simulink model "TorqueVectoring"  (R2023b)
settings: Solver=VariableStepAuto  StartTime=0.0  StopTime=25  FixedStep=1e-3  RelTol=1e-1  AbsTol=1e-3
libraries: simulink x7, autolibshared x5, fuzblock x5, vehdynlibviscommon x1, sim3dlib x1, sim3dautolib x1
(part 6 of 6)

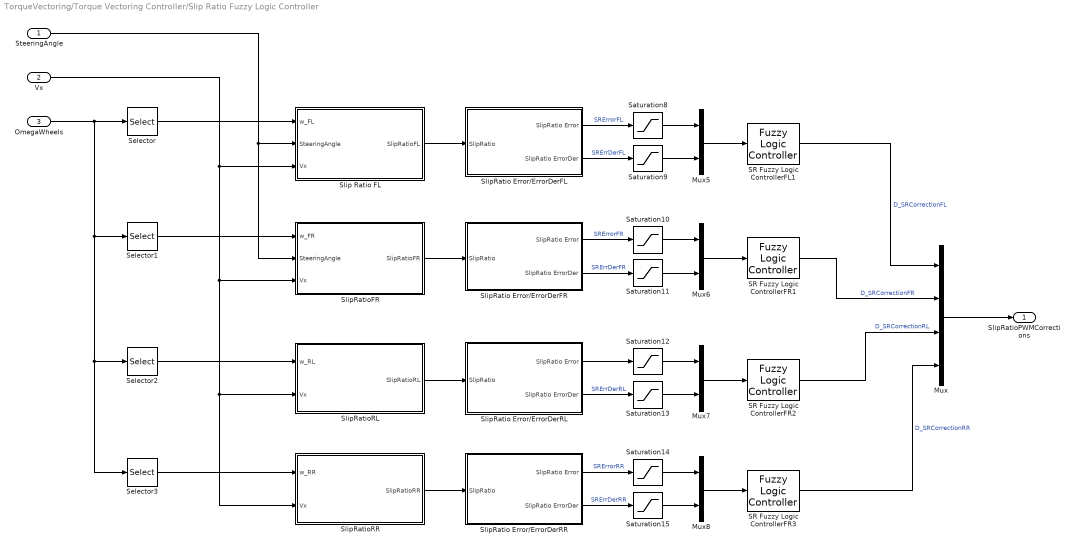
== system TorqueVectoring/Torque Vectoring Controller/Slip Ratio Fuzzy Logic Controller ==
  SteeringAngle : Inport
  Vx : Inport  Port=2
  OmegaWheels : Inport  Port=3
  Mux : Mux
  Mux{5..8} (4 alike) : Mux  Inputs=2
  SR Fuzzy Logic ControllerFL1 : fuzblock/Fuzzy Logic  Controller  FIS='SRfuzzyrules.fis'  OutputSampleNumber=101  DataType=double  FuzzifiedInputs=off  RuleFiringStrengths=off  RuleOutputs=off  AggregatedOutputs=off  SimulateUsing=Interpreted execution  OutOfRangeInputValueMessage=warning  NoRuleFiredMessage=warning  EmptyOutputFuzzySetMessage=warning
  SR Fuzzy Logic ControllerFR1 : fuzblock/Fuzzy Logic  Controller  FIS='SRfuzzyrules.fis'  OutputSampleNumber=101  DataType=double  FuzzifiedInputs=off  RuleFiringStrengths=off  RuleOutputs=off  AggregatedOutputs=off  SimulateUsing=Interpreted execution  OutOfRangeInputValueMessage=warning  NoRuleFiredMessage=warning  EmptyOutputFuzzySetMessage=warning
  SR Fuzzy Logic ControllerFR2 : fuzblock/Fuzzy Logic  Controller  FIS='SRfuzzyrules.fis'  OutputSampleNumber=101  DataType=double  FuzzifiedInputs=off  RuleFiringStrengths=off  RuleOutputs=off  AggregatedOutputs=off  SimulateUsing=Interpreted execution  OutOfRangeInputValueMessage=warning  NoRuleFiredMessage=warning  EmptyOutputFuzzySetMessage=warning
  SR Fuzzy Logic ControllerFR3 : fuzblock/Fuzzy Logic  Controller  FIS='SRfuzzyrules.fis'  OutputSampleNumber=101  DataType=double  FuzzifiedInputs=off  RuleFiringStrengths=off  RuleOutputs=off  AggregatedOutputs=off  SimulateUsing=Interpreted execution  OutOfRangeInputValueMessage=warning  NoRuleFiredMessage=warning  EmptyOutputFuzzySetMessage=warning
  Saturation{8,10,12,14} (4 alike) : Saturate  UpperLimit=30  LowerLimit=-30
  Saturation{9,11,13,15} (4 alike) : Saturate  UpperLimit=3e4  LowerLimit=-3e4
  Selector : Selector  InputPortWidth=4  IndexOptions=Index vector (dialog)  Indices=1  OutputSizes=1
  Selector1 : Selector  InputPortWidth=4  IndexOptions=Index vector (dialog)  Indices=2  OutputSizes=1
  Selector2 : Selector  InputPortWidth=4  IndexOptions=Index vector (dialog)  Indices=3  OutputSizes=1
  Selector3 : Selector  InputPortWidth=4  IndexOptions=Index vector (dialog)  Indices=4  OutputSizes=1
  Slip Ratio FL : Subsystem
  SlipRatio Error/ErrorDerFL : Subsystem
  SlipRatio Error/ErrorDerFR : Subsystem
  SlipRatio Error/ErrorDerRL : Subsystem
  SlipRatio Error/ErrorDerRR : Subsystem
  SlipRatioFR : Subsystem
  SlipRatioRL : Subsystem
  SlipRatioRR : Subsystem
  SlipRatioPWMCorrections : Outport
  wires:
  Selector/1 -> Slip Ratio FL/1(w_FL)
  Selector1/1 -> SlipRatioFR/1(w_FR)
  Selector2/1 -> SlipRatioRL/1(w_RL)
  Selector3/1 -> SlipRatioRR/1(w_RR)
  Mux/1 -> SlipRatioPWMCorrections/1
  SteeringAngle/1 -> SlipRatioFR/2(SteeringAngle), Slip Ratio FL/2(SteeringAngle)
  Vx/1 -> SlipRatioRR/2(Vx), SlipRatioRL/2(Vx), SlipRatioFR/3(Vx), Slip Ratio FL/3(Vx)
  OmegaWheels/1 -> Selector3/1, Selector2/1, Selector1/1, Selector/1
  Slip Ratio FL/1(SlipRatioFL) -> SlipRatio Error/ErrorDerFL/1(SlipRatio)
  SlipRatioFR/1(SlipRatioFR) -> SlipRatio Error/ErrorDerFR/1(SlipRatio)
  SlipRatioRL/1(SlipRatioRL) -> SlipRatio Error/ErrorDerRL/1(SlipRatio)
  SlipRatioRR/1(SlipRatioRR) -> SlipRatio Error/ErrorDerRR/1(SlipRatio)
  Saturation9/1 -> Mux5/2
  Saturation8/1 -> Mux5/1
  Mux5/1 -> SR Fuzzy Logic ControllerFL1/1
  SR Fuzzy Logic ControllerFL1/1 -> Mux/1  "D_SRCorrectionFL"
  Mux6/1 -> SR Fuzzy Logic ControllerFR1/1
  Saturation10/1 -> Mux6/1
  Saturation11/1 -> Mux6/2
  SR Fuzzy Logic ControllerFR1/1 -> Mux/2  "D_SRCorrectionFR"
  Saturation13/1 -> Mux7/2
  Saturation12/1 -> Mux7/1
  Mux7/1 -> SR Fuzzy Logic ControllerFR2/1
  SR Fuzzy Logic ControllerFR2/1 -> Mux/3  "D_SRCorrectionRL"
  Mux8/1 -> SR Fuzzy Logic ControllerFR3/1
  Saturation14/1 -> Mux8/1
  Saturation15/1 -> Mux8/2
  SR Fuzzy Logic ControllerFR3/1 -> Mux/4  "D_SRCorrectionRR"
  SlipRatio Error/ErrorDerFL/1(SlipRatio Error) -> Saturation8/1  "SRErrorFL"
  SlipRatio Error/ErrorDerFL/2(SlipRatio ErrorDer) -> Saturation9/1  "SRErrDerFL"
  SlipRatio Error/ErrorDerFR/1(SlipRatio Error) -> Saturation10/1  "SRErrorFR"
  SlipRatio Error/ErrorDerFR/2(SlipRatio ErrorDer) -> Saturation11/1  "SRErrDerFR"
  SlipRatio Error/ErrorDerRL/1(SlipRatio Error) -> Saturation12/1
  SlipRatio Error/ErrorDerRL/2(SlipRatio ErrorDer) -> Saturation13/1  "SRErrDerRL"
  SlipRatio Error/ErrorDerRR/1(SlipRatio Error) -> Saturation14/1  "SRErrorRR"
  SlipRatio Error/ErrorDerRR/2(SlipRatio ErrorDer) -> Saturation15/1  "SRErrDerRR"

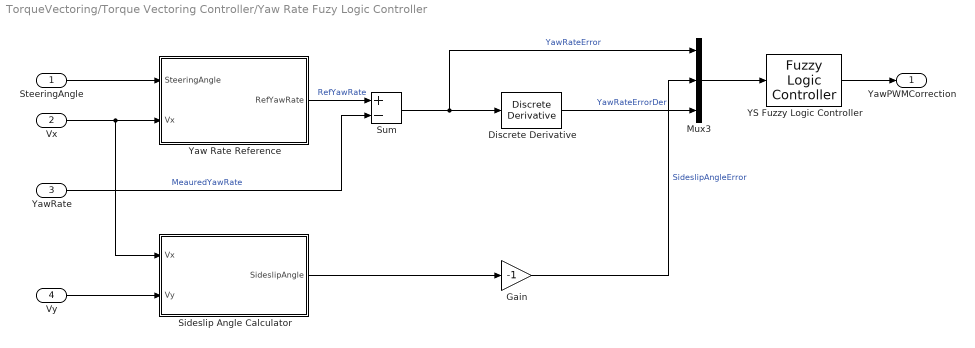
== system TorqueVectoring/Torque Vectoring Controller/Yaw Rate Fuzy Logic Controller ==
  SteeringAngle : Inport
  Vx : Inport  Port=2
  YawRate : Inport  Port=3
  Vy : Inport  Port=4
  Discrete Derivative : simulink/Discrete/Discrete Derivative  gainval=1.0  ICPrevScaledInput=0.0  OutMin=[]  OutMax=[]  OutDataType=fixdt(1, 16)  OutScaling=2^-10  DoSatur=off
  Gain : Gain  Gain=-1
  Mux3 : Mux  Inputs=3
  Sideslip Angle Calculator : Subsystem
  Sum : Sum  Inputs=+-
  YS Fuzzy Logic Controller : fuzblock/Fuzzy Logic  Controller  FIS='YSfuzzyrules.fis'  OutputSampleNumber=101  DataType=double  FuzzifiedInputs=off  RuleFiringStrengths=off  RuleOutputs=off  AggregatedOutputs=off  SimulateUsing=Interpreted execution  OutOfRangeInputValueMessage=warning  NoRuleFiredMessage=warning  EmptyOutputFuzzySetMessage=warning
  Yaw Rate Reference : Subsystem
  YawPWMCorrection : Outport
  wires:
  SteeringAngle/1 -> Yaw Rate Reference/1(SteeringAngle)
  YawRate/1 -> Sum/2  "MeauredYawRate"
  Sum/1 -> Discrete Derivative/1, Mux3/1  "YawRateError"
  Yaw Rate Reference/1(RefYawRate) -> Sum/1  "RefYawRate"
  Vx/1 -> Sideslip Angle Calculator/1(Vx), Yaw Rate Reference/2(Vx)
  Gain/1 -> Mux3/2  "SideslipAngleError"
  Discrete Derivative/1 -> Mux3/3  "YawRateErrorDer"
  Mux3/1 -> YS Fuzzy Logic Controller/1
  YS Fuzzy Logic Controller/1 -> YawPWMCorrection/1
  Vy/1 -> Sideslip Angle Calculator/2(Vy)
  Sideslip Angle Calculator/1(SideslipAngle) -> Gain/1

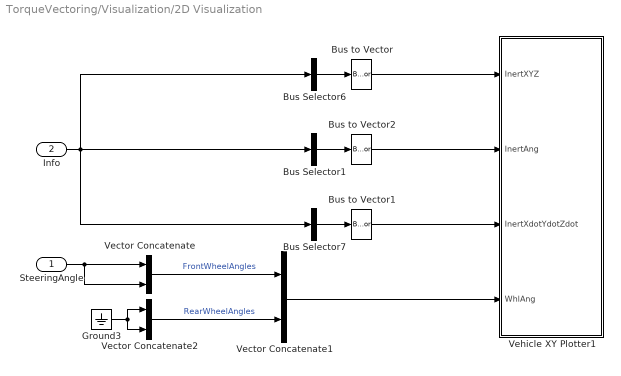
== system TorqueVectoring/Visualization/2D Visualization ==
  SteeringAngle : Inport
  Info : Inport  Port=2
  Bus Selector1 : BusSelector  OutputSignals=InertFrm.Cg.Ang.phi,InertFrm.Cg.Ang.theta,InertFrm.Cg.Ang.psi  OutputAsBus=on
  Bus Selector6 : BusSelector  OutputSignals=InertFrm.Geom.Disp.X,InertFrm.Geom.Disp.Y,InertFrm.Geom.Disp.Z  OutputAsBus=on
  Bus Selector7 : BusSelector  OutputSignals=InertFrm.Geom.Vel.Xdot,InertFrm.Geom.Vel.Ydot,InertFrm.Geom.Vel.Zdot  OutputAsBus=on
  Bus to Vector : BusToVector
  Bus to Vector1 : BusToVector
  Bus to Vector2 : BusToVector
  Ground3 : Ground
  Vector Concatenate : Concatenate
  Vector Concatenate1 : Concatenate
  Vector Concatenate2 : Concatenate
  Vehicle XY Plotter1 : Subsystem  mask(Vehicle XY Plotter){extRef=off, extStats=off, extTireF=off, a=0.175, b=0.175, w=0.2, figBorder=3, bufferSize=1024, velNorm=5, tireFNorm=1000, pltDT=0.2}
      mask prompts: extRef "Plot path reference, extRef"; extStats "Display speed, RPM and Gear"; extTireF "Display tire forces"; a "Distance to front axle from CG, a [m]:"; b "Distance to rear axle from CG, b [m]:"; w "Track width, w [m]:"; figBorder "Distance to figure borders, figBorder [m]:"; bufferSize "Path buffer sampe size, bufferSize []:"; velNorm "Velocity vector scaling, velNorm [m*s/m]:"; tireFNorm "Tire force vector scaling, tireFNorm [m/N]:"; pltDT "Plot update rate, pltDT [s]:"
      mask help:
      | This block will display a MATLAB figure which indicates the vehicle path, current position and heading velocity.
      | An optional path reference is also provided.
      mask init:
      | block = gcb;
      | if autoblkschecksimstopped(block)
      |     ParamNames = {'extRef';'extStats';'extTireF';'extTireF'};
      |     PortNames = {'RefXYZ';'Stats';'TireFx';'TireFy'};
      |     for idx=1:length(PortNames)
      |         InportOption  = {'built-in/Ground', [PortNames{idx}, ' Ground'];...
      |             'built-in/Inport',PortNames{idx}};
      |         if ~strcmp(get_param(block,ParamNames{idx}),'on')
      |             NewBlkHdl = autoblksreplaceblock(block, InportOption, 1);
      |             set_param(NewBlkHdl, 'ShowName', 'off');
      |         else
      |             autoblksreplaceblock(block, InportOption, 2);
      |         end
      |     end
      |     InportNames = {'InertXYZ';'InertAng';'InertXdotYdotZdot';'WhlAng';'RefXYZ';'Stats';'TireFx';'TireFy'};
      |     FoundNames = get_param(find_system(block, 'LookUnderMasks', 'all', 'SearchDepth', 1, 'FollowLinks', 'on', 'BlockType', 'Inport'), 'Name');
      |     [~,PortI] = intersect(InportNames, FoundNames);
      |     PortI = sort(PortI);
      |     for idx = 1:length(PortI)
      |         set_param([block, '/', InportNames{PortI(idx)}], 'Port', num2str(idx));
      |     end
      | end
      mask TypeOptions a: Vehicle XY Plotter/a
      mask TypeOptions b: Vehicle XY Plotter/b
      mask TypeOptions w: Vehicle XY Plotter/w
      mask TypeOptions figBorder: Vehicle XY Plotter/figBorder
      mask TypeOptions bufferSize: Vehicle XY Plotter/bufferSize
      mask TypeOptions velNorm: Vehicle XY Plotter/velNorm
      mask TypeOptions tireFNorm: Vehicle XY Plotter/tireFNorm
      mask DialogControl Container3 Prompt: Plot and Display Options
  wires:
  Vector Concatenate1/1 -> Vehicle XY Plotter1/4(WhlAng)
  Ground3/1 -> Vector Concatenate2/1, Vector Concatenate2/2
  Bus Selector6/1 -> Bus to Vector/1
  Vector Concatenate/1 -> Vector Concatenate1/1  "FrontWheelAngles"
  SteeringAngle/1 -> Vector Concatenate/2, Vector Concatenate/1
  Vector Concatenate2/1 -> Vector Concatenate1/2  "RearWheelAngles"
  Bus Selector7/1 -> Bus to Vector1/1
  Bus to Vector1/1 -> Vehicle XY Plotter1/3(InertXdotYdotZdot)
  Bus to Vector/1 -> Vehicle XY Plotter1/1(InertXYZ)
  Bus to Vector2/1 -> Vehicle XY Plotter1/2(InertAng)
  Bus Selector1/1 -> Bus to Vector2/1
  Info/1 -> Bus Selector6/1, Bus Selector7/1, Bus Selector1/1

== system TorqueVectoring/Plant/Wheel Front Left/DC Motor ==
  PWMVoltage : Inport
  w : Inport  Port=2
  Multiply : Gain  Gain=0.00402273
  Multiply1 : Gain  Gain=0.00006835
  Subtract : Sum  Inputs=+-
  Torque : Outport
  wires:
  Multiply1/1 -> Subtract/2
  PWMVoltage/1 -> Multiply/1
  Multiply/1 -> Subtract/1
  Subtract/1 -> Torque/1
  w/1 -> Multiply1/1

== system TorqueVectoring/Plant/Wheel Front Right/DC Motor ==
  PWMVoltage : Inport
  w : Inport  Port=2
  Multiply : Gain  Gain=0.00402273
  Multiply1 : Gain  Gain=0.00006835
  Subtract : Sum  Inputs=+-
  Torque : Outport
  wires:
  Multiply1/1 -> Subtract/2
  PWMVoltage/1 -> Multiply/1
  Multiply/1 -> Subtract/1
  Subtract/1 -> Torque/1
  w/1 -> Multiply1/1

== system TorqueVectoring/Plant/Wheel Rear Left/DC Motor ==
  PWMVoltage : Inport
  w : Inport  Port=2
  Multiply : Gain  Gain=0.00402273
  Multiply1 : Gain  Gain=0.00006835
  Subtract : Sum  Inputs=+-
  Torque : Outport
  wires:
  Multiply1/1 -> Subtract/2
  PWMVoltage/1 -> Multiply/1
  Multiply/1 -> Subtract/1
  Subtract/1 -> Torque/1
  w/1 -> Multiply1/1

== system TorqueVectoring/Plant/Wheel Rear Right/DC Motor ==
  PWMVoltage : Inport
  w : Inport  Port=2
  Multiply : Gain  Gain=0.00402273
  Multiply1 : Gain  Gain=0.00006835
  Subtract : Sum  Inputs=+-
  Torque : Outport
  wires:
  Multiply1/1 -> Subtract/2
  PWMVoltage/1 -> Multiply/1
  Multiply/1 -> Subtract/1
  Subtract/1 -> Torque/1
  w/1 -> Multiply1/1

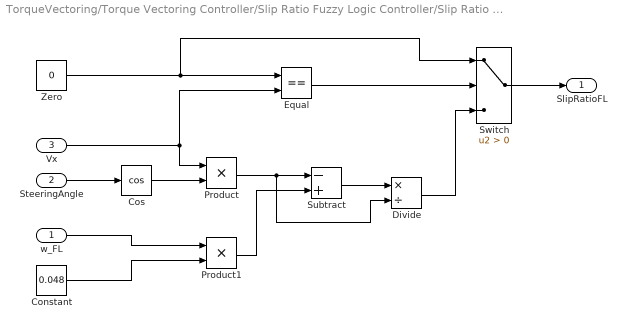
== system TorqueVectoring/Torque Vectoring Controller/Slip Ratio Fuzzy Logic Controller/Slip Ratio FL ==
  w_FL : Inport
  SteeringAngle : Inport  Port=2
  Vx : Inport  Port=3
  Constant : Constant  Value=0.048
  Cos : Trigonometry  Operator=cos
  Divide : Product  Inputs=*/
  Equal : RelationalOperator  Operator===  OutDataTypeStr=boolean  RndMeth=Simplest  InputSameDT=off
  Product : Product
  Product1 : Product
  Subtract : Sum  Inputs=-+
  Switch : Switch  Criteria=u2 > Threshold  SaturateOnIntegerOverflow=off  InputSameDT=off
  Zero : Constant  Value=0  OutDataTypeStr=Inherit: Inherit via back propagation
  SlipRatioFL : Outport
  wires:
  Constant/1 -> Product1/2
  SteeringAngle/1 -> Cos/1
  Product/1 -> Divide/2, Subtract/1
  Product1/1 -> Subtract/2
  Subtract/1 -> Divide/1
  Cos/1 -> Product/2
  w_FL/1 -> Product1/1
  Vx/1 -> Equal/2, Product/1
  Zero/1 -> Switch/1, Equal/1
  Equal/1 -> Switch/2
  Switch/1 -> SlipRatioFL/1
  Divide/1 -> Switch/3

== system TorqueVectoring/Torque Vectoring Controller/Slip Ratio Fuzzy Logic Controller/SlipRatio Error//ErrorDerFL ==
  SlipRatio : Inport
  Discrete Derivative : simulink/Discrete/Discrete Derivative  gainval=1.0  ICPrevScaledInput=0.0  OutMin=[]  OutMax=[]  OutDataType=fixdt(1, 16)  OutScaling=2^-10  DoSatur=off
  SlipRatioError1 : Sum  Inputs=+-
  SlipRatioRef1 : Subsystem
  SlipRatioToError1 : Subsystem
  SlipRatio Error : Outport
  SlipRatio ErrorDer : Outport  Port=2
  wires:
  SlipRatioToError1/1(SlipRatioToError) -> SlipRatioError1/2  "D_SRactual"
  SlipRatioRef1/1(SlipRatioRef) -> SlipRatioError1/1  "D_SRref"
  SlipRatioError1/1 -> SlipRatio Error/1, Discrete Derivative/1
  SlipRatio/1 -> SlipRatioToError1/1(SlipRatio), SlipRatioRef1/1(SlipRatio)
  Discrete Derivative/1 -> SlipRatio ErrorDer/1

== system TorqueVectoring/Torque Vectoring Controller/Slip Ratio Fuzzy Logic Controller/SlipRatio Error//ErrorDerFR ==
  SlipRatio : Inport
  Discrete Derivative1 : simulink/Discrete/Discrete Derivative  gainval=1.0  ICPrevScaledInput=0.0  OutMin=[]  OutMax=[]  OutDataType=fixdt(1, 16)  OutScaling=2^-10  DoSatur=off
  SlipRatioError1 : Sum  Inputs=+-
  SlipRatioRef1 : Subsystem
  SlipRatioToError1 : Subsystem
  SlipRatio Error : Outport
  SlipRatio ErrorDer : Outport  Port=2
  wires:
  SlipRatio/1 -> SlipRatioToError1/1(SlipRatio), SlipRatioRef1/1(SlipRatio)
  SlipRatioToError1/1(SlipRatioToError) -> SlipRatioError1/2  "D_SRactual"
  SlipRatioRef1/1(SlipRatioRef) -> SlipRatioError1/1  "D_SRrefFR"
  Discrete Derivative1/1 -> SlipRatio ErrorDer/1
  SlipRatioError1/1 -> SlipRatio Error/1, Discrete Derivative1/1

== system TorqueVectoring/Torque Vectoring Controller/Slip Ratio Fuzzy Logic Controller/SlipRatio Error//ErrorDerRL ==
  SlipRatio : Inport
  Discrete Derivative1 : simulink/Discrete/Discrete Derivative  gainval=1.0  ICPrevScaledInput=0.0  OutMin=[]  OutMax=[]  OutDataType=fixdt(1, 16)  OutScaling=2^-10  DoSatur=off
  SlipRatioError1 : Sum  Inputs=+-
  SlipRatioRef1 : Subsystem
  SlipRatioToError1 : Subsystem
  SlipRatio Error : Outport
  SlipRatio ErrorDer : Outport  Port=2
  wires:
  SlipRatioRef1/1(SlipRatioRef) -> SlipRatioError1/1  "D_SRrefRL"
  SlipRatioError1/1 -> SlipRatio Error/1, Discrete Derivative1/1
  SlipRatio/1 -> SlipRatioToError1/1(SlipRatio), SlipRatioRef1/1(SlipRatio)
  Discrete Derivative1/1 -> SlipRatio ErrorDer/1
  SlipRatioToError1/1(SlipRatioToError) -> SlipRatioError1/2  "D_SRactual"

== system TorqueVectoring/Torque Vectoring Controller/Slip Ratio Fuzzy Logic Controller/SlipRatio Error//ErrorDerRR ==
  SlipRatio : Inport
  Discrete Derivative1 : simulink/Discrete/Discrete Derivative  gainval=1.0  ICPrevScaledInput=0.0  OutMin=[]  OutMax=[]  OutDataType=fixdt(1, 16)  OutScaling=2^-10  DoSatur=off
  SlipRatioError1 : Sum  Inputs=+-
  SlipRatioRef1 : Subsystem
  SlipRatioToError1 : Subsystem
  SlipRatio Error : Outport
  SlipRatio ErrorDer : Outport  Port=2
  wires:
  SlipRatioToError1/1(SlipRatioToError) -> SlipRatioError1/2  "D_SRactual"
  SlipRatio/1 -> SlipRatioToError1/1(SlipRatio), SlipRatioRef1/1(SlipRatio)
  Discrete Derivative1/1 -> SlipRatio ErrorDer/1
  SlipRatioRef1/1(SlipRatioRef) -> SlipRatioError1/1  "D_SRrefRR"
  SlipRatioError1/1 -> SlipRatio Error/1, Discrete Derivative1/1

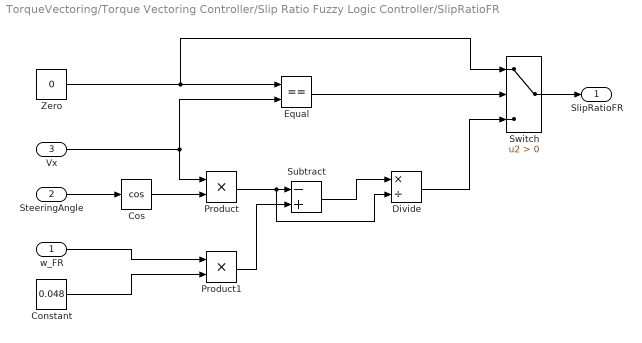
== system TorqueVectoring/Torque Vectoring Controller/Slip Ratio Fuzzy Logic Controller/SlipRatioFR ==
  w_FR : Inport
  SteeringAngle : Inport  Port=2
  Vx : Inport  Port=3
  Constant : Constant  Value=0.048
  Cos : Trigonometry  Operator=cos
  Divide : Product  Inputs=*/
  Equal : RelationalOperator  Operator===  OutDataTypeStr=boolean  RndMeth=Simplest  InputSameDT=off
  Product : Product
  Product1 : Product
  Subtract : Sum  Inputs=-+
  Switch : Switch  Criteria=u2 > Threshold  SaturateOnIntegerOverflow=off  InputSameDT=off
  Zero : Constant  Value=0  OutDataTypeStr=Inherit: Inherit via back propagation
  SlipRatioFR : Outport
  wires:
  w_FR/1 -> Product1/1
  Cos/1 -> Product/2
  Subtract/1 -> Divide/1
  Product1/1 -> Subtract/2
  Product/1 -> Subtract/1, Divide/2
  SteeringAngle/1 -> Cos/1
  Constant/1 -> Product1/2
  Vx/1 -> Equal/2, Product/1
  Switch/1 -> SlipRatioFR/1
  Divide/1 -> Switch/3
  Zero/1 -> Switch/1, Equal/1
  Equal/1 -> Switch/2

== system TorqueVectoring/Torque Vectoring Controller/Slip Ratio Fuzzy Logic Controller/SlipRatioRL ==
  w_RL : Inport
  Vx : Inport  Port=2
  Constant : Constant  Value=0.048
  Divide : Product  Inputs=*/
  Equal : RelationalOperator  Operator===  OutDataTypeStr=boolean  RndMeth=Simplest  InputSameDT=off
  Product1 : Product
  Subtract : Sum  Inputs=-+
  Switch : Switch  Criteria=u2 > Threshold  SaturateOnIntegerOverflow=off  InputSameDT=off
  Zero : Constant  Value=0  OutDataTypeStr=Inherit: Inherit via back propagation
  SlipRatioRL : Outport
  wires:
  Constant/1 -> Product1/2
  Product1/1 -> Subtract/2
  Subtract/1 -> Divide/1
  w_RL/1 -> Product1/1
  Vx/1 -> Equal/2, Divide/2, Subtract/1
  Divide/1 -> Switch/3
  Zero/1 -> Switch/1, Equal/1
  Equal/1 -> Switch/2
  Switch/1 -> SlipRatioRL/1

== system TorqueVectoring/Torque Vectoring Controller/Slip Ratio Fuzzy Logic Controller/SlipRatioRR ==
  w_RR : Inport
  Vx : Inport  Port=2
  Constant : Constant  Value=0.048
  Divide : Product  Inputs=*/
  Equal : RelationalOperator  Operator===  OutDataTypeStr=boolean  RndMeth=Simplest  InputSameDT=off
  Product1 : Product
  Subtract : Sum  Inputs=-+
  Switch : Switch  Criteria=u2 > Threshold  SaturateOnIntegerOverflow=off  InputSameDT=off
  Zero : Constant  Value=0  OutDataTypeStr=Inherit: Inherit via back propagation
  SlipRatioRR : Outport
  wires:
  w_RR/1 -> Product1/1
  Subtract/1 -> Divide/1
  Product1/1 -> Subtract/2
  Constant/1 -> Product1/2
  Vx/1 -> Equal/2, Subtract/1, Divide/2
  Divide/1 -> Switch/3
  Zero/1 -> Switch/1, Equal/1
  Equal/1 -> Switch/2
  Switch/1 -> SlipRatioRR/1

== system TorqueVectoring/Torque Vectoring Controller/Yaw Rate Fuzy Logic Controller/Sideslip Angle Calculator ==
  Vx : Inport
  Vy : Inport  Port=2
  Atan : Trigonometry  Operator=atan
  Divide : Product  Inputs=*/
  Equal : RelationalOperator  Operator===  OutDataTypeStr=boolean  RndMeth=Simplest  InputSameDT=off
  Switch : Switch  Criteria=u2 > Threshold  SaturateOnIntegerOverflow=off  InputSameDT=off
  Zero : Constant  Value=0  OutDataTypeStr=Inherit: Inherit via back propagation
  SideslipAngle : Outport
  wires:
  Divide/1 -> Atan/1
  Vx/1 -> Equal/2, Divide/2
  Vy/1 -> Divide/1
  Equal/1 -> Switch/2
  Zero/1 -> Switch/1, Equal/1
  Switch/1 -> SideslipAngle/1
  Atan/1 -> Switch/3

== system TorqueVectoring/Torque Vectoring Controller/Yaw Rate Fuzy Logic Controller/Yaw Rate Reference ==
  SteeringAngle : Inport
  Vx : Inport  Port=2
  Constant : Constant  Value=0.23
  Divide : Product  Inputs=*/
  Product : Product
  Tan : Trigonometry  Operator=tan
  RefYawRate : Outport
  wires:
  Product/1 -> Divide/1
  Vx/1 -> Product/2
  Constant/1 -> Divide/2
  SteeringAngle/1 -> Tan/1
  Tan/1 -> Product/1
  Divide/1 -> RefYawRate/1

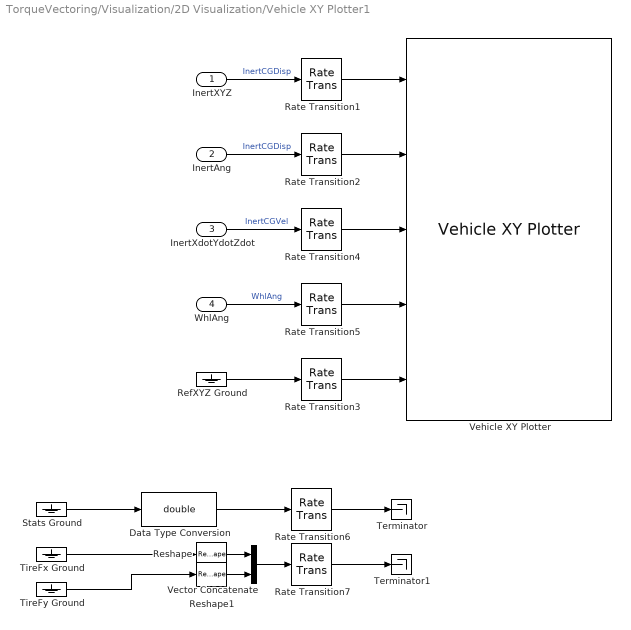
== system TorqueVectoring/Visualization/2D Visualization/Vehicle XY Plotter1 ==
  InertXYZ : Inport
  InertAng : Inport  Port=2
  InertXdotYdotZdot : Inport  Port=3
  WhlAng : Inport  Port=4
  Data Type Conversion : DataTypeConversion  OutDataTypeStr=double  SaturateOnIntegerOverflow=off  RndMeth=Floor
  Rate Transition{1..7} (7 alike) : RateTransition  Deterministic=off  OutPortSampleTime=pltDT
  RefXYZ Ground : Ground
  Reshape : Reshape  OutputDimensionality=Row vector (2-D)
  Reshape1 : Reshape  OutputDimensionality=Row vector (2-D)
  Stats Ground : Ground
  Terminator : Terminator
  Terminator1 : Terminator
  TireFx Ground : Ground
  TireFy Ground : Ground
  Vector Concatenate : Concatenate  Mode=Multidimensional array
  Vehicle XY Plotter : vehdynlibviscommon/Vehicle XY Plotter  w=w  a=a  b=b  figBorder=figBorder  bufferSize=bufferSize  extStats=off  extTireF=off
  wires:
  Vector Concatenate/1 -> Rate Transition7/1
  Reshape1/1 -> Vector Concatenate/2
  Reshape/1 -> Vector Concatenate/1
  Rate Transition7/1 -> Terminator1/1
  Data Type Conversion/1 -> Rate Transition6/1
  Rate Transition6/1 -> Terminator/1
  Rate Transition5/1 -> Vehicle XY Plotter/4
  Rate Transition4/1 -> Vehicle XY Plotter/3
  Rate Transition2/1 -> Vehicle XY Plotter/2
  Rate Transition1/1 -> Vehicle XY Plotter/1
  Rate Transition3/1 -> Vehicle XY Plotter/5
  WhlAng/1 -> Rate Transition5/1  "WhlAng"
  InertXYZ/1 -> Rate Transition1/1  "InertCGDisp"
  InertXdotYdotZdot/1 -> Rate Transition4/1  "InertCGVel"
  InertAng/1 -> Rate Transition2/1  "InertCGDisp"
  RefXYZ Ground/1 -> Rate Transition3/1
  Stats Ground/1 -> Data Type Conversion/1
  TireFx Ground/1 -> Reshape/1
  TireFy Ground/1 -> Reshape1/1

== system TorqueVectoring/Torque Vectoring Controller/Slip Ratio Fuzzy Logic Controller/SlipRatio Error//ErrorDerFL/SlipRatioRef1 ==
  SlipRatio : Inport
  If : If  IfExpression=u1 >= 0
  If Action Subsystem : Subsystem  TreatAsAtomicUnit=on
  If Action Subsystem1 : Subsystem  TreatAsAtomicUnit=on
  Merge : Merge
  SlipRatioRef : Outport
  wires:
  SlipRatio/1 -> If/1
  Merge/1 -> SlipRatioRef/1
  If Action Subsystem/1(Out1) -> Merge/1
  If Action Subsystem1/1(Out1) -> Merge/2
  If/2 -> If Action Subsystem1/Action
  If/1 -> If Action Subsystem/Action

== system TorqueVectoring/Torque Vectoring Controller/Slip Ratio Fuzzy Logic Controller/SlipRatio Error//ErrorDerFL/SlipRatioToError1 ==
  SlipRatio : Inport
  If : If  IfExpression=u1 > 0.1 | u1 < -0.1  ElseIfExpressions=u1 <= 0.1 & u1 >= 0, u1 >= -0.1 & u1 < 0  ShowElse=off
  If Action Subsystem : Subsystem  TreatAsAtomicUnit=on
  If Action Subsystem1 : Subsystem  TreatAsAtomicUnit=on
  If Action Subsystem2 : Subsystem  TreatAsAtomicUnit=on
  Merge : Merge  Inputs=3
  SlipRatioToError : Outport
  wires:
  If Action Subsystem1/1(Out1) -> Merge/2
  SlipRatio/1 -> If/1, If Action Subsystem/1(SlipRatio)
  If Action Subsystem2/1(Out1) -> Merge/3
  If/1 -> If Action Subsystem/Action
  If/2 -> If Action Subsystem1/Action
  If Action Subsystem/1(Out1) -> Merge/1
  Merge/1 -> SlipRatioToError/1
  If/3 -> If Action Subsystem2/Action

== system TorqueVectoring/Torque Vectoring Controller/Slip Ratio Fuzzy Logic Controller/SlipRatio Error//ErrorDerFR/SlipRatioRef1 ==
  SlipRatio : Inport
  If : If  IfExpression=u1 >= 0
  If Action Subsystem : Subsystem  TreatAsAtomicUnit=on
  If Action Subsystem1 : Subsystem  TreatAsAtomicUnit=on
  Merge : Merge
  SlipRatioRef : Outport
  wires:
  SlipRatio/1 -> If/1
  Merge/1 -> SlipRatioRef/1
  If Action Subsystem/1(Out1) -> Merge/1
  If Action Subsystem1/1(Out1) -> Merge/2
  If/2 -> If Action Subsystem1/Action
  If/1 -> If Action Subsystem/Action

== system TorqueVectoring/Torque Vectoring Controller/Slip Ratio Fuzzy Logic Controller/SlipRatio Error//ErrorDerFR/SlipRatioToError1 ==
  SlipRatio : Inport
  If : If  IfExpression=u1 > 0.1 | u1 < -0.1  ElseIfExpressions=u1 <= 0.1 & u1 >= 0, u1 >= -0.1 & u1 < 0  ShowElse=off
  If Action Subsystem : Subsystem  TreatAsAtomicUnit=on
  If Action Subsystem1 : Subsystem  TreatAsAtomicUnit=on
  If Action Subsystem2 : Subsystem  TreatAsAtomicUnit=on
  Merge : Merge  Inputs=3
  SlipRatioToError : Outport
  wires:
  If Action Subsystem1/1(Out1) -> Merge/2
  SlipRatio/1 -> If/1, If Action Subsystem/1(SlipRatio)
  If Action Subsystem2/1(Out1) -> Merge/3
  If/1 -> If Action Subsystem/Action
  If/2 -> If Action Subsystem1/Action
  If Action Subsystem/1(Out1) -> Merge/1
  Merge/1 -> SlipRatioToError/1
  If/3 -> If Action Subsystem2/Action

== system TorqueVectoring/Torque Vectoring Controller/Slip Ratio Fuzzy Logic Controller/SlipRatio Error//ErrorDerRL/SlipRatioRef1 ==
  SlipRatio : Inport
  If : If  IfExpression=u1 >= 0
  If Action Subsystem : Subsystem  TreatAsAtomicUnit=on
  If Action Subsystem1 : Subsystem  TreatAsAtomicUnit=on
  Merge : Merge
  SlipRatioRef : Outport
  wires:
  SlipRatio/1 -> If/1
  Merge/1 -> SlipRatioRef/1
  If Action Subsystem/1(Out1) -> Merge/1
  If Action Subsystem1/1(Out1) -> Merge/2
  If/2 -> If Action Subsystem1/Action
  If/1 -> If Action Subsystem/Action

== system TorqueVectoring/Torque Vectoring Controller/Slip Ratio Fuzzy Logic Controller/SlipRatio Error//ErrorDerRL/SlipRatioToError1 ==
  SlipRatio : Inport
  If : If  IfExpression=u1 > 0.1 | u1 < -0.1  ElseIfExpressions=u1 <= 0.1 & u1 >= 0, u1 >= -0.1 & u1 < 0  ShowElse=off
  If Action Subsystem : Subsystem  TreatAsAtomicUnit=on
  If Action Subsystem1 : Subsystem  TreatAsAtomicUnit=on
  If Action Subsystem2 : Subsystem  TreatAsAtomicUnit=on
  Merge : Merge  Inputs=3
  SlipRatioToError : Outport
  wires:
  If Action Subsystem1/1(Out1) -> Merge/2
  SlipRatio/1 -> If/1, If Action Subsystem/1(SlipRatio)
  If Action Subsystem2/1(Out1) -> Merge/3
  If/1 -> If Action Subsystem/Action
  If/2 -> If Action Subsystem1/Action
  If Action Subsystem/1(Out1) -> Merge/1
  Merge/1 -> SlipRatioToError/1
  If/3 -> If Action Subsystem2/Action

== system TorqueVectoring/Torque Vectoring Controller/Slip Ratio Fuzzy Logic Controller/SlipRatio Error//ErrorDerRR/SlipRatioRef1 ==
  SlipRatio : Inport
  If : If  IfExpression=u1 >= 0
  If Action Subsystem : Subsystem  TreatAsAtomicUnit=on
  If Action Subsystem1 : Subsystem  TreatAsAtomicUnit=on
  Merge : Merge
  SlipRatioRef : Outport
  wires:
  SlipRatio/1 -> If/1
  Merge/1 -> SlipRatioRef/1
  If Action Subsystem/1(Out1) -> Merge/1
  If Action Subsystem1/1(Out1) -> Merge/2
  If/2 -> If Action Subsystem1/Action
  If/1 -> If Action Subsystem/Action

== system TorqueVectoring/Torque Vectoring Controller/Slip Ratio Fuzzy Logic Controller/SlipRatio Error//ErrorDerRR/SlipRatioToError1 ==
  SlipRatio : Inport
  If : If  IfExpression=u1 > 0.1 | u1 < -0.1  ElseIfExpressions=u1 <= 0.1 & u1 >= 0, u1 >= -0.1 & u1 < 0  ShowElse=off
  If Action Subsystem : Subsystem  TreatAsAtomicUnit=on
  If Action Subsystem1 : Subsystem  TreatAsAtomicUnit=on
  If Action Subsystem2 : Subsystem  TreatAsAtomicUnit=on
  Merge : Merge  Inputs=3
  SlipRatioToError : Outport
  wires:
  If Action Subsystem1/1(Out1) -> Merge/2
  SlipRatio/1 -> If/1, If Action Subsystem/1(SlipRatio)
  If Action Subsystem2/1(Out1) -> Merge/3
  If/1 -> If Action Subsystem/Action
  If/2 -> If Action Subsystem1/Action
  If Action Subsystem/1(Out1) -> Merge/1
  Merge/1 -> SlipRatioToError/1
  If/3 -> If Action Subsystem2/Action

== system TorqueVectoring/Torque Vectoring Controller/Slip Ratio Fuzzy Logic Controller/SlipRatio Error//ErrorDerFL/SlipRatioRef1/If Action Subsystem ==
  Action Port : ActionPort  ActionPortLabel=if(u1 >= 0)
  Constant : Constant  Value=0.1
  Out1 : Outport
  wires:
  Constant/1 -> Out1/1

== system TorqueVectoring/Torque Vectoring Controller/Slip Ratio Fuzzy Logic Controller/SlipRatio Error//ErrorDerFL/SlipRatioRef1/If Action Subsystem1 ==
  Action Port : ActionPort  ActionPortLabel=else
  Constant : Constant  Value=-0.1
  Out1 : Outport
  wires:
  Constant/1 -> Out1/1

== system TorqueVectoring/Torque Vectoring Controller/Slip Ratio Fuzzy Logic Controller/SlipRatio Error//ErrorDerFL/SlipRatioToError1/If Action Subsystem ==
  SlipRatio : Inport
  Action Port : ActionPort  ActionPortLabel=if(u1 > 0.1 | u1 < -0.1)
  Out1 : Outport
  wires:
  SlipRatio/1 -> Out1/1

== system TorqueVectoring/Torque Vectoring Controller/Slip Ratio Fuzzy Logic Controller/SlipRatio Error//ErrorDerFL/SlipRatioToError1/If Action Subsystem1 ==
  Action Port : ActionPort  ActionPortLabel=elseif( u1 <= 0.1 & u1 >= 0)
  Constant : Constant  Value=0.1
  Out1 : Outport
  wires:
  Constant/1 -> Out1/1

== system TorqueVectoring/Torque Vectoring Controller/Slip Ratio Fuzzy Logic Controller/SlipRatio Error//ErrorDerFL/SlipRatioToError1/If Action Subsystem2 ==
  Action Port : ActionPort  ActionPortLabel=elseif( u1 >= -0.1 & u1 < 0)
  Constant : Constant  Value=-0.1
  Out1 : Outport
  wires:
  Constant/1 -> Out1/1

== system TorqueVectoring/Torque Vectoring Controller/Slip Ratio Fuzzy Logic Controller/SlipRatio Error//ErrorDerFR/SlipRatioRef1/If Action Subsystem ==
  Action Port : ActionPort  ActionPortLabel=if(u1 >= 0)
  Constant : Constant  Value=0.1
  Out1 : Outport
  wires:
  Constant/1 -> Out1/1

== system TorqueVectoring/Torque Vectoring Controller/Slip Ratio Fuzzy Logic Controller/SlipRatio Error//ErrorDerFR/SlipRatioRef1/If Action Subsystem1 ==
  Action Port : ActionPort  ActionPortLabel=else
  Constant : Constant  Value=-0.1
  Out1 : Outport
  wires:
  Constant/1 -> Out1/1

== system TorqueVectoring/Torque Vectoring Controller/Slip Ratio Fuzzy Logic Controller/SlipRatio Error//ErrorDerFR/SlipRatioToError1/If Action Subsystem ==
  SlipRatio : Inport
  Action Port : ActionPort  ActionPortLabel=if(u1 > 0.1 | u1 < -0.1)
  Out1 : Outport
  wires:
  SlipRatio/1 -> Out1/1

== system TorqueVectoring/Torque Vectoring Controller/Slip Ratio Fuzzy Logic Controller/SlipRatio Error//ErrorDerFR/SlipRatioToError1/If Action Subsystem1 ==
  Action Port : ActionPort  ActionPortLabel=elseif( u1 <= 0.1 & u1 >= 0)
  Constant : Constant  Value=0.1
  Out1 : Outport
  wires:
  Constant/1 -> Out1/1

== system TorqueVectoring/Torque Vectoring Controller/Slip Ratio Fuzzy Logic Controller/SlipRatio Error//ErrorDerFR/SlipRatioToError1/If Action Subsystem2 ==
  Action Port : ActionPort  ActionPortLabel=elseif( u1 >= -0.1 & u1 < 0)
  Constant : Constant  Value=-0.1
  Out1 : Outport
  wires:
  Constant/1 -> Out1/1

== system TorqueVectoring/Torque Vectoring Controller/Slip Ratio Fuzzy Logic Controller/SlipRatio Error//ErrorDerRL/SlipRatioRef1/If Action Subsystem ==
  Action Port : ActionPort  ActionPortLabel=if(u1 >= 0)
  Constant : Constant  Value=0.1
  Out1 : Outport
  wires:
  Constant/1 -> Out1/1

== system TorqueVectoring/Torque Vectoring Controller/Slip Ratio Fuzzy Logic Controller/SlipRatio Error//ErrorDerRL/SlipRatioRef1/If Action Subsystem1 ==
  Action Port : ActionPort  ActionPortLabel=else
  Constant : Constant  Value=-0.1
  Out1 : Outport
  wires:
  Constant/1 -> Out1/1

== system TorqueVectoring/Torque Vectoring Controller/Slip Ratio Fuzzy Logic Controller/SlipRatio Error//ErrorDerRL/SlipRatioToError1/If Action Subsystem ==
  SlipRatio : Inport
  Action Port : ActionPort  ActionPortLabel=if(u1 > 0.1 | u1 < -0.1)
  Out1 : Outport
  wires:
  SlipRatio/1 -> Out1/1

== system TorqueVectoring/Torque Vectoring Controller/Slip Ratio Fuzzy Logic Controller/SlipRatio Error//ErrorDerRL/SlipRatioToError1/If Action Subsystem1 ==
  Action Port : ActionPort  ActionPortLabel=elseif( u1 <= 0.1 & u1 >= 0)
  Constant : Constant  Value=0.1
  Out1 : Outport
  wires:
  Constant/1 -> Out1/1

== system TorqueVectoring/Torque Vectoring Controller/Slip Ratio Fuzzy Logic Controller/SlipRatio Error//ErrorDerRL/SlipRatioToError1/If Action Subsystem2 ==
  Action Port : ActionPort  ActionPortLabel=elseif( u1 >= -0.1 & u1 < 0)
  Constant : Constant  Value=-0.1
  Out1 : Outport
  wires:
  Constant/1 -> Out1/1

== system TorqueVectoring/Torque Vectoring Controller/Slip Ratio Fuzzy Logic Controller/SlipRatio Error//ErrorDerRR/SlipRatioRef1/If Action Subsystem ==
  Action Port : ActionPort  ActionPortLabel=if(u1 >= 0)
  Constant : Constant  Value=0.1
  Out1 : Outport
  wires:
  Constant/1 -> Out1/1

== system TorqueVectoring/Torque Vectoring Controller/Slip Ratio Fuzzy Logic Controller/SlipRatio Error//ErrorDerRR/SlipRatioRef1/If Action Subsystem1 ==
  Action Port : ActionPort  ActionPortLabel=else
  Constant : Constant  Value=-0.1
  Out1 : Outport
  wires:
  Constant/1 -> Out1/1

== system TorqueVectoring/Torque Vectoring Controller/Slip Ratio Fuzzy Logic Controller/SlipRatio Error//ErrorDerRR/SlipRatioToError1/If Action Subsystem ==
  SlipRatio : Inport
  Action Port : ActionPort  ActionPortLabel=if(u1 > 0.1 | u1 < -0.1)
  Out1 : Outport
  wires:
  SlipRatio/1 -> Out1/1

== system TorqueVectoring/Torque Vectoring Controller/Slip Ratio Fuzzy Logic Controller/SlipRatio Error//ErrorDerRR/SlipRatioToError1/If Action Subsystem1 ==
  Action Port : ActionPort  ActionPortLabel=elseif( u1 <= 0.1 & u1 >= 0)
  Constant : Constant  Value=0.1
  Out1 : Outport
  wires:
  Constant/1 -> Out1/1

== system TorqueVectoring/Torque Vectoring Controller/Slip Ratio Fuzzy Logic Controller/SlipRatio Error//ErrorDerRR/SlipRatioToError1/If Action Subsystem2 ==
  Action Port : ActionPort  ActionPortLabel=elseif( u1 >= -0.1 & u1 < 0)
  Constant : Constant  Value=-0.1
  Out1 : Outport
  wires:
  Constant/1 -> Out1/1
